simulink model "Quadrotor_simulation"  (R2019a)
settings: Solver=ode4  StartTime=0.0  StopTime=P.tsim  FixedStep=0.01  RelTol=1e-3
InitFcn:
  | Parameters
undefined symbols (not defined in the file or in its folder): Att_Head_PD_ctrl, Att_heading_MST_SMC, Att_heading_SMC, Dist_att, Dist_att2, Dist_pos, E_Kalman_Filter, GPS, IMU, LPF, LPF_F, P, Position_MST_SMC, Position_PD_Ctrl, Position_SMC, Quad_states_plot, Quadrotor_draw, Trajectory
settings Model: Creator=Hp_lap  LastModifiedBy=User
settings SolverCC: AlgebraicLoopSolver=LineSearch
settings DataIOCC: SaveFormat=Array  SaveState=on  DSMLogging=off  ReturnWorkspaceOutputs=off  LoggingToFile=on

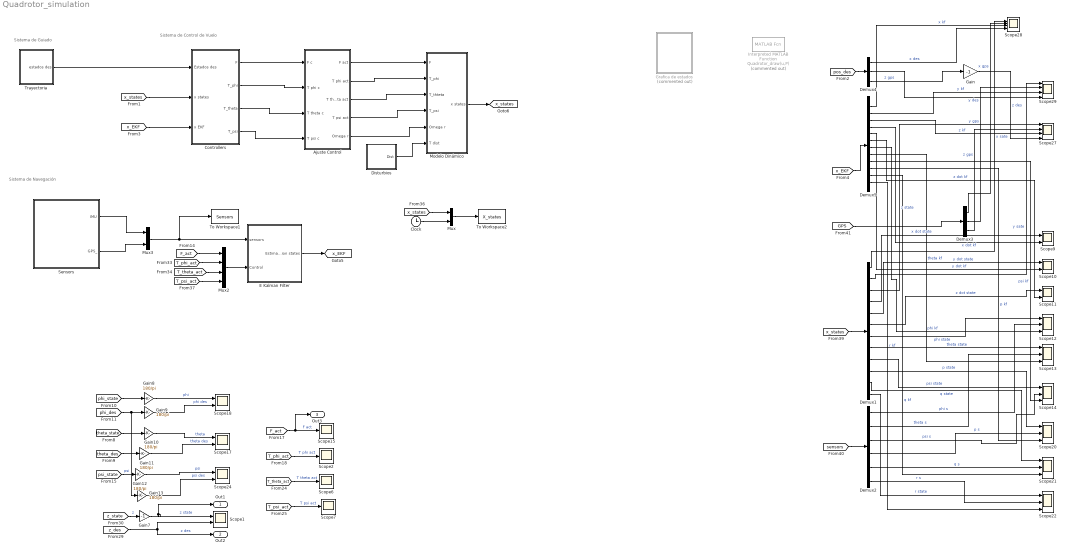
== system Quadrotor_simulation ==
  note: Sistema de Navegación
  note: Sistema de Control de Vuelo
  note: Sistema de Guiado
  Ajuste Control : Subsystem
  Clock : Clock
  Controllers : Subsystem
  Demux1 : Demux  Outputs=12
  Demux2 : Demux  Outputs=6
  Demux3 : Demux  Outputs=3
  Demux4 : Demux  Outputs=3
  Demux5 : Demux  Outputs=12
  Disturbios : Subsystem
  E Kalman Filter : Subsystem
  Gain : Gain  Gain=-1
  Gain{8..13} (6 alike) : Gain  Gain=180/pi
  Gain7 : Gain  Gain=-1
  Grafica de estados : Subsystem  Commented=on
  Interpreted MATLAB Function : MATLABFcn  Commented=on  MATLABFcn=Quadrotor_draw(u,P)  OutputDimensions=0  SampleTime=0.1
  Modelo Dinámico : Subsystem
  Mux : Mux  Inputs=2
  Mux2 : Mux
  Mux3 : Mux  Inputs=2
  Scope{1,9..11,17..18,24} (7 alike) : Scope  NumInputPorts=2
  Scope{12..14,20..22} (6 alike) : Scope  NumInputPorts=3
  Scope{2,6..7,15} (4 alike) : Scope
  Scope27 : Scope  NumInputPorts=4
  Scope28 : Scope  NumInputPorts=4
  Scope29 : Scope  NumInputPorts=4
  Sensors : Subsystem
  To Workspace1 : ToWorkspace  VariableName=Sensors  SampleTime=0.01
  To Workspace2 : ToWorkspace  VariableName=X_states  SampleTime=0.01
  Trayectoria : Subsystem
  Out1 : Outport
  Out2 : Outport  Port=2
  Out3 : Outport  Port=3
  tag scope: x_EKF=global, x_states=global
  wires:
  Mux/1 -> To Workspace2/1
  Clock/1 -> Mux/2
  Disturbios/1(Dist) -> Modelo Dinámico/6(T dist)
  [x_states] -> Mux/1
  Demux5/1 -> Scope28/3  "x kf"
  Demux5/2 -> Scope29/3  "y kf"
  Demux5/3 -> Scope27/3  "z kf"
  Demux5/4 -> Scope9/2  "x dot kf"
  Demux5/5 -> Scope10/2  "y dot kf"
  Demux5/6 -> Scope11/2  "z dot kf"
  Demux5/10 -> Scope20/3  "p kf"
  Demux5/11 -> Scope21/3  "q kf"
  Demux5/12 -> Scope22/3  "r kf"
  [GPS] -> Demux3/1
  Demux1/3 -> Scope27/1  "z state"
  Demux1/1 -> Scope28/1  "x sate"
  Demux3/1 -> Scope28/2  "x gps"
  Demux1/2 -> Scope29/1  "y sate"
  Demux3/2 -> Scope29/2  "y gps"
  Demux3/3 -> Scope27/2  "z gps"
  [x_states] -> Demux1/1
  [sensors] -> Demux2/1
  Demux1/4 -> Scope9/1  "x dot state"
  Demux1/5 -> Scope10/1  "y dot state"
  Demux1/6 -> Scope11/1  "z dot state"
  Demux1/7 -> Scope12/1  "phi state"
  Demux5/7 -> Scope12/3  "phi kf"
  Demux2/1 -> Scope12/2  "phi s"
  Demux1/8 -> Scope13/1  "theta state"
  Demux2/2 -> Scope13/2  "theta s"
  Demux1/9 -> Scope14/1  "psi state"
  Demux2/3 -> Scope14/2  "psi s"
  Demux5/8 -> Scope13/3  "theta kf"
  Demux5/9 -> Scope14/3  "psi kf"
  Demux1/10 -> Scope20/1  "p state"
  Demux2/4 -> Scope20/2  "p s"
  Demux1/11 -> Scope21/1  "q state"
  Demux2/5 -> Scope21/2  "q s"
  Demux1/12 -> Scope22/1  "r state"
  Demux2/6 -> Scope22/2  "r s"
  Modelo Dinámico/1(x states) -> [x_states]
  [pos_des] -> Demux4/1
  Demux4/3 -> Gain/1  "z gps"
  Gain/1 -> Scope27/4  "z des"
  Demux4/2 -> Scope29/4  "y des"
  Demux4/1 -> Scope28/4  "x des"
  Ajuste Control/5(Omega r) -> Modelo Dinámico/5(Omega r)
  [x_states] -> Controllers/2(" x states")
  [x_EKF] -> Controllers/3(x EKF)
  Gain12/1 -> Scope24/1  "psi"
  [psi_state] -> Gain12/1  "psi"
  [theta_des] -> Gain11/1
  Gain9/1 -> Scope18/2  "phi des"
  [phi_des] -> Gain13/1, Gain9/1
  [theta_state] -> Gain10/1
  Gain11/1 -> Scope17/2  "theta des"
  Gain13/1 -> Scope24/2  "psi des"
  Gain8/1 -> Scope18/1  "phi"
  Gain10/1 -> Scope17/1  "theta"
  [phi_state] -> Gain8/1
  [z_des] -> Scope1/2, Out2/1  "z des"
  Gain7/1 -> Scope1/1, Out1/1  "z state"
  [z_state] -> Gain7/1  "z"
  Controllers/1(F) -> Ajuste Control/1(F c)
  Controllers/2(T_phi) -> Ajuste Control/2(T phi c)
  Controllers/3(T_theta) -> Ajuste Control/3(T theta c)
  Controllers/4(T_psi) -> Ajuste Control/4(T psi c)
  [F_act] -> Out3/1, Scope15/1  "F act"
  [T_phi_act] -> Scope2/1  "T phi act"
  [T_theta_act] -> Scope6/1  "T theta act"
  [T_psi_act] -> Scope7/1  "T psi act"
  Ajuste Control/1(F act) -> Modelo Dinámico/1(F)
  Ajuste Control/2(T phi act) -> Modelo Dinámico/2(T_phi)
  Ajuste Control/3(T theta act) -> Modelo Dinámico/3(T_thteta)
  Ajuste Control/4(T psi act) -> Modelo Dinámico/4(T_psi)
  [T_phi_act] -> Mux2/2
  [F_act] -> Mux2/1
  Sensors/2(GPS_) -> Mux3/2
  Sensors/1(IMU) -> Mux3/1
  [T_psi_act] -> Mux2/4
  E Kalman Filter/1(Estimation states) -> [x_EKF]
  [T_theta_act] -> Mux2/3
  Mux2/1 -> E Kalman Filter/2(Control)
  Mux3/1 -> To Workspace1/1, E Kalman Filter/1(sensors)
  [x_EKF] -> Demux5/1
  Trayectoria/1("\testados des") -> Controllers/1(Estados des)

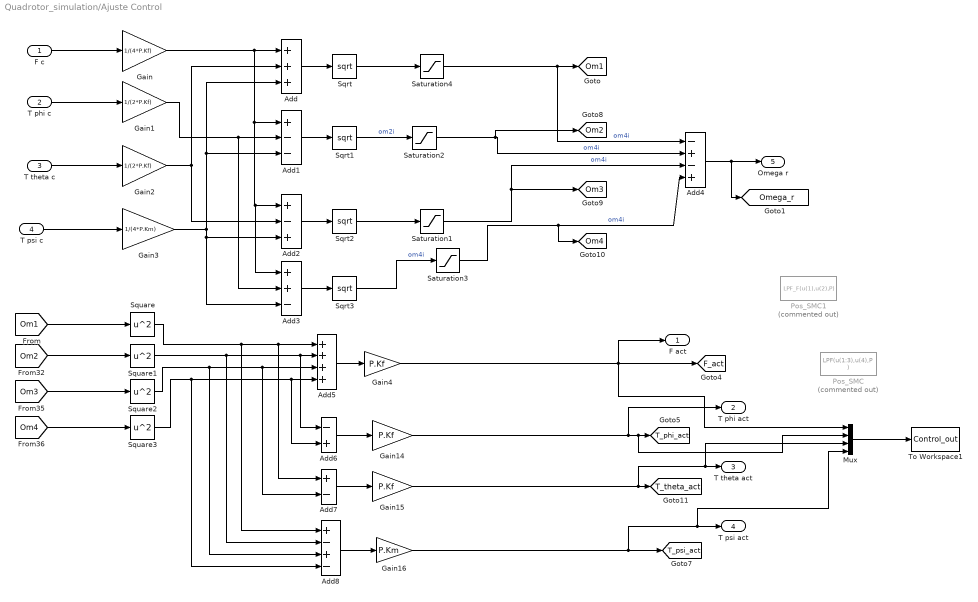
== system Quadrotor_simulation/Ajuste Control ==
  F c : Inport
  T phi c : Inport  Port=2
  T theta c : Inport  Port=3
  T psi c : Inport  Port=4
  Add : Sum  Inputs=+++
  Add1 : Sum  Inputs=+--
  Add2 : Sum  Inputs=+-+
  Add3 : Sum  Inputs=++-
  Add4 : Sum  Inputs=-+-+
  Add5 : Sum  Inputs=++++
  Add6 : Sum  Inputs=-+
  Add7 : Sum  Inputs=+-
  Add8 : Sum  Inputs=+-+-
  Gain : Gain  Gain=1/(4*P.Kf)
  Gain1 : Gain  Gain=1/(2*P.Kf)
  Gain14 : Gain  Gain=P.Kf
  Gain15 : Gain  Gain=P.Kf
  Gain16 : Gain  Gain=P.Km
  Gain2 : Gain  Gain=1/(2*P.Kf)
  Gain3 : Gain  Gain=1/(4*P.Km)
  Gain4 : Gain  Gain=P.Kf
  Mux : Mux
  Pos_SMC : MATLABFcn  Commented=on  MATLABFcn=LPF(u(1:3),u(4),P )  OutputDimensions=3  SampleTime=0.01
  Pos_SMC1 : MATLABFcn  Commented=on  MATLABFcn=LPF_F(u(1),u(2),P)  OutputDimensions=1  SampleTime=0.01
  Saturation{1..4} (4 alike) : Saturate  UpperLimit=435  LowerLimit=0
  Sqrt{,1..3} (4 alike) : Sqrt  OutputSignalType=real  SaturateOnIntegerOverflow=on
  Square{,1..3} (4 alike) : Math  Operator=square  SaturateOnIntegerOverflow=on
  To Workspace1 : ToWorkspace  VariableName=Control_out  SampleTime=0.01
  F act : Outport
  T phi act : Outport  Port=2
  T theta act : Outport  Port=3
  T psi act : Outport  Port=4
  Omega r : Outport  Port=5
  tag scope: F_act=global, Om1=global, Om2=global, Om3=global, Om4=global, Omega_r=global, T_phi_act=global, T_psi_act=global, T_theta_act=global
  wires:
  Add4/1 -> [Omega_r], Omega r/1
  Square2/1 -> Add8/3, Add7/2, Add5/3
  Add8/1 -> Gain16/1
  Gain/1 -> Add/1, Add3/1, Add2/1, Add1/1
  Square/1 -> Add8/1, Add7/1, Add5/1
  Gain1/1 -> Add1/2, Add3/2
  Gain3/1 -> Add3/3, Add2/3, Add1/3, Add/3
  Gain2/1 -> Add2/2, Add/2
  Square1/1 -> Add8/2, Add6/1, Add5/2
  Add/1 -> Sqrt/1
  Add6/1 -> Gain14/1
  Add1/1 -> Sqrt1/1
  Add2/1 -> Sqrt2/1
  [Om1] -> Square/1
  Add5/1 -> Gain4/1
  [Om2] -> Square1/1
  Add3/1 -> Sqrt3/1
  [Om3] -> Square2/1
  Square3/1 -> Add8/4, Add6/2, Add5/4
  Add7/1 -> Gain15/1
  [Om4] -> Square3/1
  Mux/1 -> To Workspace1/1
  Gain16/1 -> Mux/4, T psi act/1, [T_psi_act]
  Gain15/1 -> Mux/3, T theta act/1, [T_theta_act]
  Gain14/1 -> T phi act/1, Mux/2, [T_phi_act]
  Gain4/1 -> F act/1, [F_act], Mux/1
  Sqrt3/1 -> Saturation3/1  "om4i"
  Saturation3/1 -> [Om4], Add4/4  "om4i"
  Sqrt2/1 -> Saturation1/1
  Saturation1/1 -> Add4/3, [Om3]  "om4i"
  Sqrt1/1 -> Saturation2/1  "om2i"
  Saturation2/1 -> [Om2], Add4/2  "om4i"
  Sqrt/1 -> Saturation4/1
  Saturation4/1 -> Add4/1, [Om1]  "om4i"
  F c/1 -> Gain/1
  T phi c/1 -> Gain1/1
  T theta c/1 -> Gain2/1
  T psi c/1 -> Gain3/1

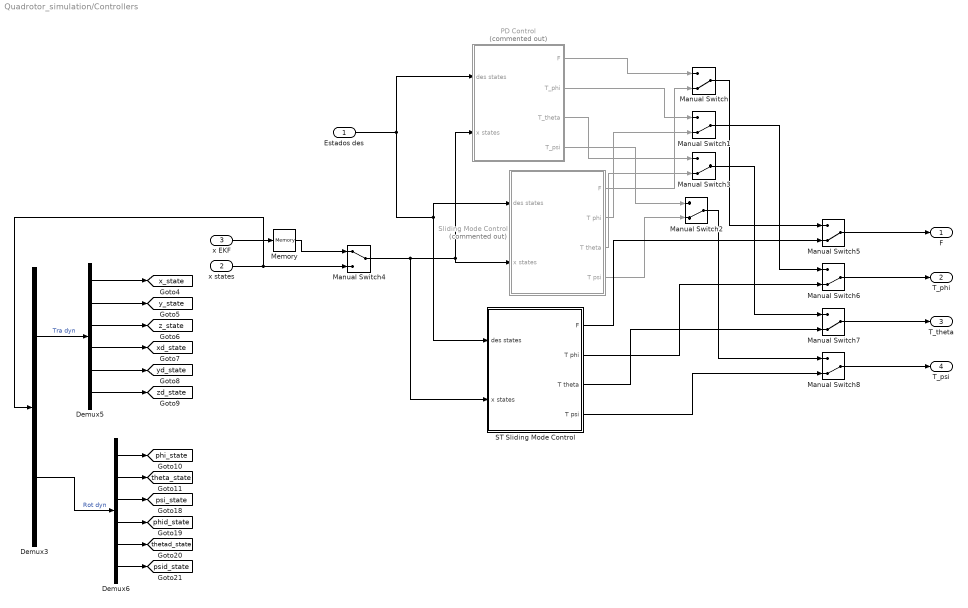
== system Quadrotor_simulation/Controllers ==
  Estados des : Inport
  " x states" : Inport  Port=2
  x EKF : Inport  Port=3
  Demux3 : Demux  Outputs=2
  Demux5 : Demux  Outputs=6
  Demux6 : Demux  Outputs=6
  Manual Switch{,1..3,5..8} (8 alike) : ManualSwitch  CurrentSetting=0
  Manual Switch4 : ManualSwitch
  Memory : Memory  InitialCondition=[P.x0;P.y0;P.z0;P.x0_dot;P.y0_dot;P.z0_dot;P.phi0;P.theta0;P.psi0;P.phi0_dot;P.theta0_dot;P.psi0_dot]  LinearizeMemory=on  LinearizeAsDelay=on
  PD Control : Subsystem  Commented=on
  "ST Sliding Mode Control " : Subsystem
  "Sliding Mode Control " : Subsystem  Commented=on
  F : Outport
  T_phi : Outport  Port=2
  T_theta : Outport  Port=3
  T_psi : Outport  Port=4
  tag scope: phi_state=global, phid_state=global, psi_state=global, psid_state=global, theta_state=global, thetad_state=global, x_state=global, xd_state=global, y_state=global, yd_state=global, z_state=global, zd_state=global
  wires:
  "Sliding Mode Control "/1(F) -> Manual Switch/2
  "Sliding Mode Control "/2(T phi) -> Manual Switch1/2
  "Sliding Mode Control "/3(T theta) -> Manual Switch3/2
  "Sliding Mode Control "/4(T psi) -> Manual Switch2/2
  x EKF/1 -> Memory/1
  Manual Switch4/1 -> "ST Sliding Mode Control "/2(x states), "Sliding Mode Control "/2(x states), PD Control/2(x states)
  Memory/1 -> Manual Switch4/1
  Estados des/1 -> PD Control/1(des states), "ST Sliding Mode Control "/1(des states), "Sliding Mode Control "/1(des states)
  PD Control/1(F) -> Manual Switch/1
  PD Control/2(T_phi) -> Manual Switch1/1
  PD Control/3(T_theta) -> Manual Switch3/1
  PD Control/4(T_psi) -> Manual Switch2/1
  Manual Switch/1 -> Manual Switch5/1
  Manual Switch1/1 -> Manual Switch6/1
  Manual Switch3/1 -> Manual Switch7/1
  Manual Switch2/1 -> Manual Switch8/1
  Demux5/6 -> [zd_state]
  Demux6/6 -> [psid_state]
  Demux6/5 -> [thetad_state]
  Demux6/4 -> [phid_state]
  Demux3/1 -> Demux5/1  "Tra dyn"
  Demux3/2 -> Demux6/1  "Rot dyn"
  Demux6/3 -> [psi_state]
  Demux5/1 -> [x_state]
  Demux5/3 -> [z_state]
  Demux6/2 -> [theta_state]
  Demux5/2 -> [y_state]
  Demux5/5 -> [yd_state]
  Demux5/4 -> [xd_state]
  " x states"/1 -> Demux3/1, Manual Switch4/2
  Demux6/1 -> [phi_state]
  "ST Sliding Mode Control "/1(F) -> Manual Switch5/2
  "ST Sliding Mode Control "/2(T phi) -> Manual Switch6/2
  "ST Sliding Mode Control "/3(T theta) -> Manual Switch7/2
  "ST Sliding Mode Control "/4(T psi) -> Manual Switch8/2
  Manual Switch5/1 -> F/1
  Manual Switch6/1 -> T_phi/1
  Manual Switch7/1 -> T_theta/1
  Manual Switch8/1 -> T_psi/1

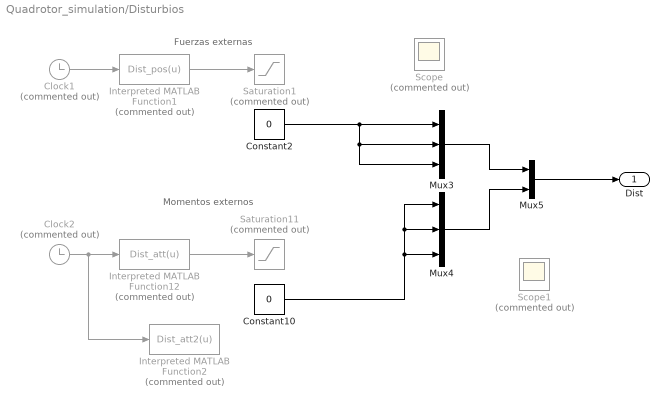
== system Quadrotor_simulation/Disturbios ==
  note: Momentos externos
  note: Fuerzas externas
  Clock1 : Clock  Commented=on
  Clock2 : Clock  Commented=on
  Constant10 : Constant  Value=0
  Constant2 : Constant  Value=0
  Interpreted MATLAB Function1 : MATLABFcn  Commented=on  MATLABFcn=Dist_pos(u)  OutputDimensions=1  SampleTime=0.01
  Interpreted MATLAB Function12 : MATLABFcn  Commented=on  MATLABFcn=Dist_att(u)  OutputDimensions=1  SampleTime=0.01
  Interpreted MATLAB Function2 : MATLABFcn  Commented=on  MATLABFcn=Dist_att2(u)  OutputDimensions=1  SampleTime=0.01
  Mux3 : Mux  Inputs=3
  Mux4 : Mux  Inputs=3
  Mux5 : Mux  Inputs=2
  Saturation1 : Saturate  Commented=on
  Saturation11 : Saturate  Commented=on  UpperLimit=0.25  LowerLimit=-0.25
  Scope : Scope  Commented=on
  Scope1 : Scope  Commented=on
  Dist : Outport
  wires:
  Interpreted MATLAB Function12/1 -> Saturation11/1
  Mux3/1 -> Mux5/1
  Mux4/1 -> Mux5/2
  Mux5/1 -> Dist/1
  Clock2/1 -> Interpreted MATLAB Function2/1, Interpreted MATLAB Function12/1
  Interpreted MATLAB Function1/1 -> Saturation1/1
  Clock1/1 -> Interpreted MATLAB Function1/1
  Constant2/1 -> Mux3/3, Mux3/2, Mux3/1
  Constant10/1 -> Mux4/3, Mux4/2, Mux4/1

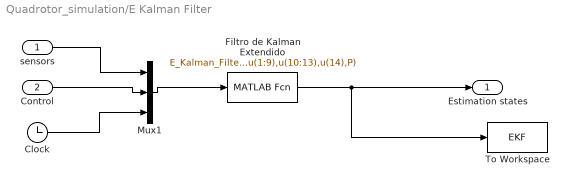
== system Quadrotor_simulation/E Kalman Filter ==
  sensors : Inport
  Control : Inport  Port=2
  Clock : Clock
  Filtro de Kalman Extendido : MATLABFcn  MATLABFcn=E_Kalman_Filter(u(1:9),u(10:13),u(14),P)  OutputDimensions=12  SampleTime=0.01
  Mux1 : Mux  Inputs=3
  To Workspace : ToWorkspace  VariableName=EKF  SampleTime=0.01
  Estimation states : Outport
  wires:
  Mux1/1 -> Filtro de Kalman Extendido/1
  Clock/1 -> Mux1/3
  Control/1 -> Mux1/2
  sensors/1 -> Mux1/1
  Filtro de Kalman Extendido/1 -> To Workspace/1, Estimation states/1

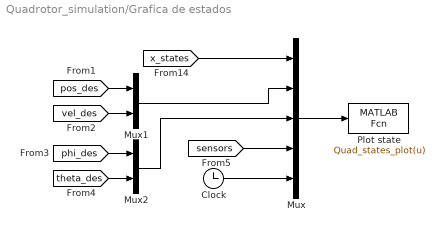
== system Quadrotor_simulation/Grafica de estados ==
  Clock : Clock
  Mux : Mux  Inputs=5
  Mux1 : Mux  Inputs=2
  Mux2 : Mux  Inputs=2
  Plot state : MATLABFcn  MATLABFcn=Quad_states_plot(u)  OutputDimensions=0  SampleTime=0.1
  wires:
  Mux/1 -> Plot state/1
  [x_states] -> Mux/1
  [vel_des] -> Mux1/2
  [pos_des] -> Mux1/1
  Mux1/1 -> Mux/2
  [theta_des] -> Mux2/2
  [phi_des] -> Mux2/1
  Mux2/1 -> Mux/3
  [sensors] -> Mux/4
  Clock/1 -> Mux/5

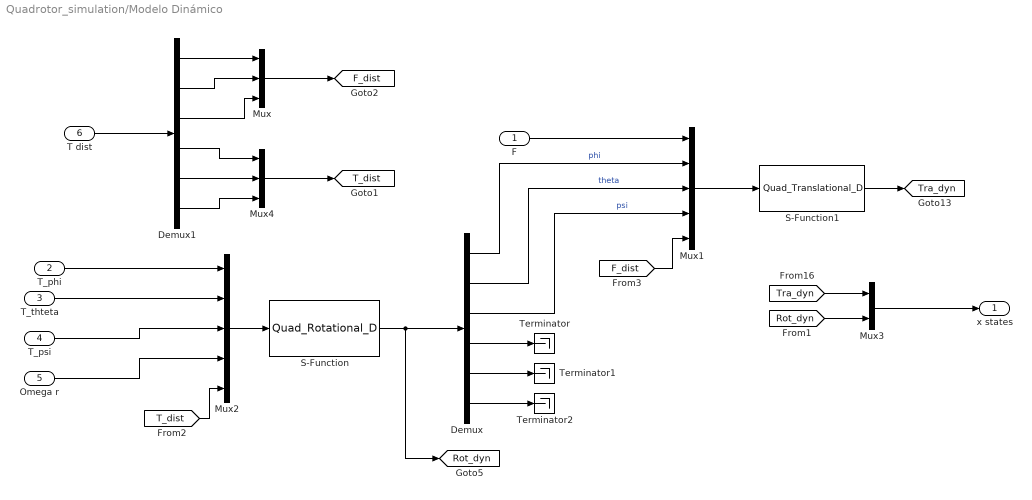
== system Quadrotor_simulation/Modelo Dinámico ==
  F : Inport
  T_phi : Inport  Port=2
  T_thteta : Inport  Port=3
  T_psi : Inport  Port=4
  Omega r : Inport  Port=5
  T dist : Inport  Port=6
  Demux : Demux  Outputs=6
  Demux1 : Demux  Outputs=6
  Mux : Mux  Inputs=3
  Mux1 : Mux  Inputs=5
  Mux2 : Mux  Inputs=5
  Mux3 : Mux  Inputs=2
  Mux4 : Mux  Inputs=3
  S-Function : S-Function  FunctionName=Quad_Rotational_D  Parameters=P  SFunctionDeploymentMode=off  EnableBusSupport=off
  S-Function1 : S-Function  InitFcn=Parameters  FunctionName=Quad_Translational_D  Parameters=P  SFunctionDeploymentMode=off  EnableBusSupport=off
  Terminator : Terminator
  Terminator1 : Terminator
  Terminator2 : Terminator
  x states : Outport
  tag scope: F_dist=global, Rot_dyn=global, T_dist=global, Tra_dyn=global
  wires:
  Mux1/1 -> S-Function1/1
  Mux2/1 -> S-Function/1
  S-Function1/1 -> [Tra_dyn]
  S-Function/1 -> [Rot_dyn], Demux/1
  Demux/2 -> Mux1/3  "theta"
  Demux/1 -> Mux1/2  "phi"
  Demux/3 -> Mux1/4  "psi"
  Demux/6 -> Terminator2/1
  Demux/5 -> Terminator1/1
  Demux/4 -> Terminator/1
  [Tra_dyn] -> Mux3/1
  [Rot_dyn] -> Mux3/2
  T dist/1 -> Demux1/1
  Demux1/1 -> Mux/1
  Demux1/2 -> Mux/2
  Demux1/3 -> Mux/3
  Demux1/4 -> Mux4/1
  Demux1/5 -> Mux4/2
  Demux1/6 -> Mux4/3
  Mux/1 -> [F_dist]
  Mux4/1 -> [T_dist]
  [T_dist] -> Mux2/5
  [F_dist] -> Mux1/5
  F/1 -> Mux1/1
  T_phi/1 -> Mux2/1
  T_thteta/1 -> Mux2/2
  T_psi/1 -> Mux2/3
  Omega r/1 -> Mux2/4
  Mux3/1 -> x states/1

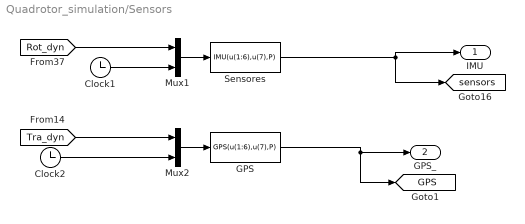
== system Quadrotor_simulation/Sensors ==
  Clock1 : Clock
  Clock2 : Clock
  GPS : MATLABFcn  MATLABFcn=GPS(u(1:6),u(7),P)  OutputDimensions=3  SampleTime=P.Ts_gps
  Mux1 : Mux  Inputs=2
  Mux2 : Mux  Inputs=2
  Sensores : MATLABFcn  MATLABFcn=IMU(u(1:6),u(7),P)  OutputDimensions=6  SampleTime=0.01
  IMU : Outport
  GPS_ : Outport  Port=2
  tag scope: GPS=global, sensors=global
  wires:
  Clock1/1 -> Mux1/2
  Mux1/1 -> Sensores/1
  Mux2/1 -> GPS/1
  Clock2/1 -> Mux2/2
  Sensores/1 -> IMU/1, [sensors]
  GPS/1 -> [GPS], GPS_/1
  [Rot_dyn] -> Mux1/1
  [Tra_dyn] -> Mux2/1

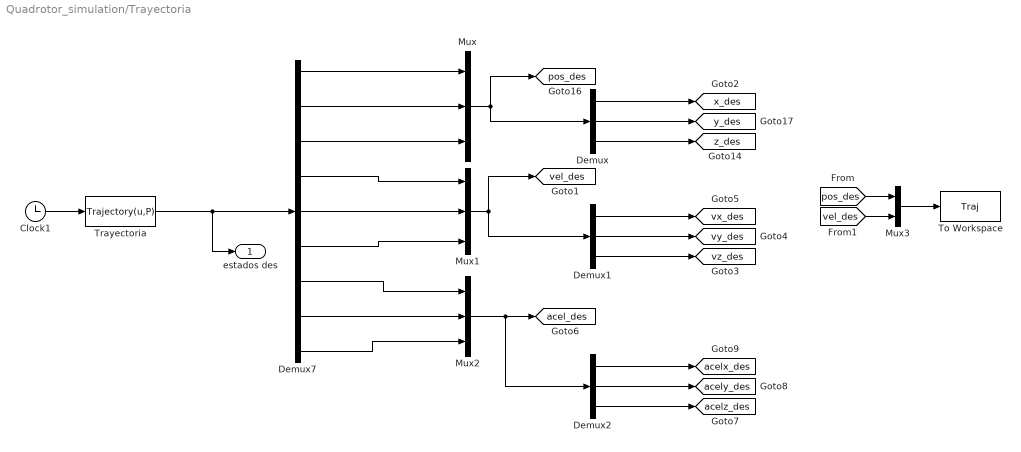
== system Quadrotor_simulation/Trayectoria ==
  Clock1 : Clock
  Demux : Demux  Outputs=3
  Demux1 : Demux  Outputs=3
  Demux2 : Demux  Outputs=3
  Demux7 : Demux  Outputs=9
  Mux : Mux  Inputs=3
  Mux1 : Mux  Inputs=3
  Mux2 : Mux  Inputs=3
  Mux3 : Mux  Inputs=2
  To Workspace : ToWorkspace  VariableName=Traj  SampleTime=0.01
  Trayectoria : MATLABFcn  MATLABFcn=Trajectory(u,P)  OutputDimensions=9  SampleTime=0.01
  "\testados des" : Outport
  tag scope: acel_des=global, acelx_des=global, acely_des=global, acelz_des=global, pos_des=global, vel_des=global, vx_des=global, vy_des=global, vz_des=global, x_des=global, y_des=global, z_des=global
  wires:
  Demux7/6 -> Mux1/3
  Demux7/4 -> Mux1/1
  Clock1/1 -> Trayectoria/1
  Demux7/1 -> Mux/1
  Demux7/5 -> Mux1/2
  Demux7/2 -> Mux/2
  Demux7/3 -> Mux/3
  Demux7/7 -> Mux2/1
  Demux7/8 -> Mux2/2
  Demux7/9 -> Mux2/3
  Mux3/1 -> To Workspace/1
  [pos_des] -> Mux3/1
  [vel_des] -> Mux3/2
  Demux/1 -> [x_des]
  Demux/3 -> [z_des]
  Demux/2 -> [y_des]
  Mux/1 -> Demux/1, [pos_des]
  Mux1/1 -> Demux1/1, [vel_des]
  Demux1/3 -> [vz_des]
  Demux1/2 -> [vy_des]
  Demux1/1 -> [vx_des]
  Demux2/1 -> [acelx_des]
  Mux2/1 -> Demux2/1, [acel_des]
  Demux2/2 -> [acely_des]
  Demux2/3 -> [acelz_des]
  Trayectoria/1 -> "\testados des"/1, Demux7/1

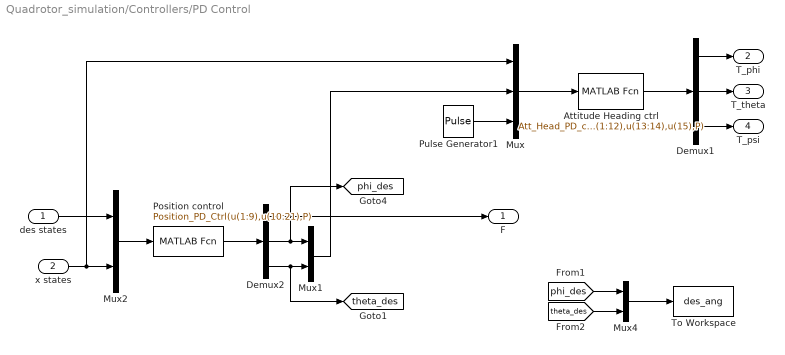
== system Quadrotor_simulation/Controllers/PD Control ==
  des states : Inport
  x states : Inport  Port=2
  Attitude Heading ctrl : MATLABFcn  MATLABFcn=Att_Head_PD_ctrl(u(1:12),u(13:14),u(15),P)  OutputDimensions=3  SampleTime=0.01
  Demux1 : Demux  Outputs=3
  Demux2 : Demux  Outputs=3
  Mux : Mux  Inputs=3
  Mux1 : Mux  Inputs=2
  Mux2 : Mux  Inputs=2
  Mux4 : Mux  Inputs=2
  Position control : MATLABFcn  MATLABFcn=Position_PD_Ctrl(u(1:9),u(10:21),P)  OutputDimensions=3  SampleTime=0.01
  Pulse Generator1 : DiscretePulseGenerator  PulseType=Time based  Amplitude=5*(pi/180)  PulseWidth=50
  To Workspace : ToWorkspace  VariableName=des_ang  SampleTime=0.01
  F : Outport
  T_phi : Outport  Port=2
  T_theta : Outport  Port=3
  T_psi : Outport  Port=4
  tag scope: phi_des=global, theta_des=global
  wires:
  Demux1/1 -> T_phi/1
  Demux1/2 -> T_theta/1
  Demux1/3 -> T_psi/1
  Attitude Heading ctrl/1 -> Demux1/1
  Mux/1 -> Attitude Heading ctrl/1
  Mux2/1 -> Position control/1
  des states/1 -> Mux2/1
  x states/1 -> Mux/1, Mux2/2
  Mux1/1 -> Mux/2
  Demux2/3 -> [theta_des], Mux1/2
  Demux2/1 -> F/1
  Position control/1 -> Demux2/1
  Mux4/1 -> To Workspace/1
  [theta_des] -> Mux4/2
  [phi_des] -> Mux4/1
  Demux2/2 -> [phi_des], Mux1/1
  Pulse Generator1/1 -> Mux/3

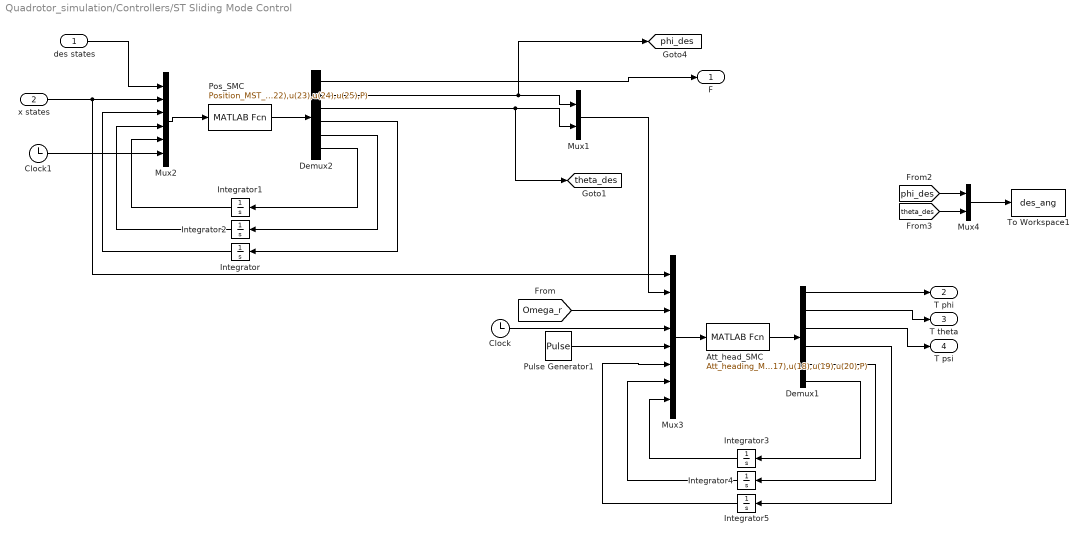
== system Quadrotor_simulation/Controllers/ST Sliding Mode Control  ==
  des states : Inport
  x states : Inport  Port=2
  Att_head_SMC : MATLABFcn  MATLABFcn=Att_heading_MST_SMC(u(1:12),u(13:14),u(15),u(16),u(17),u(18),u(19),u(20),P)  OutputDimensions=6  SampleTime=0.01
  Clock : Clock
  Clock1 : Clock
  Demux1 : Demux  Outputs=6
  Demux2 : Demux  Outputs=6
  Integrator{,1..5} (6 alike) : Integrator
  Mux1 : Mux  Inputs=2
  Mux2 : Mux  Inputs=6
  Mux3 : Mux  Inputs=8
  Mux4 : Mux  Inputs=2
  Pos_SMC : MATLABFcn  MATLABFcn=Position_MST_SMC(u(1:9),u(10:21),u(22),u(23),u(24),u(25),P)  OutputDimensions=6  SampleTime=0.01
  Pulse Generator1 : DiscretePulseGenerator  PulseType=Time based  Amplitude=5*(pi/180)  PulseWidth=50
  To Workspace1 : ToWorkspace  VariableName=des_ang  SampleTime=0.01
  F : Outport
  T phi : Outport  Port=2
  T theta : Outport  Port=3
  T psi : Outport  Port=4
  tag scope: phi_des=global, theta_des=global
  wires:
  Pos_SMC/1 -> Demux2/1
  Mux3/1 -> Att_head_SMC/1
  Att_head_SMC/1 -> Demux1/1
  Demux1/1 -> T phi/1
  Demux1/2 -> T theta/1
  Demux1/3 -> T psi/1
  des states/1 -> Mux2/1
  x states/1 -> Mux3/1, Mux2/2
  Mux2/1 -> Pos_SMC/1
  Demux2/1 -> F/1
  Demux2/2 -> [phi_des], Mux1/1
  Mux1/1 -> Mux3/2
  [Omega_r] -> Mux3/3
  Clock/1 -> Mux3/4
  Pulse Generator1/1 -> Mux3/5
  Demux2/3 -> [theta_des], Mux1/2
  Demux2/4 -> Integrator/1
  Demux2/6 -> Integrator1/1
  Demux2/5 -> Integrator2/1
  Demux1/4 -> Integrator5/1
  Demux1/5 -> Integrator4/1
  Demux1/6 -> Integrator3/1
  Mux4/1 -> To Workspace1/1
  [theta_des] -> Mux4/2
  [phi_des] -> Mux4/1
  Integrator/1 -> Mux2/3
  Integrator2/1 -> Mux2/4
  Integrator1/1 -> Mux2/5
  Integrator5/1 -> Mux3/6
  Integrator4/1 -> Mux3/7
  Integrator3/1 -> Mux3/8
  Clock1/1 -> Mux2/6

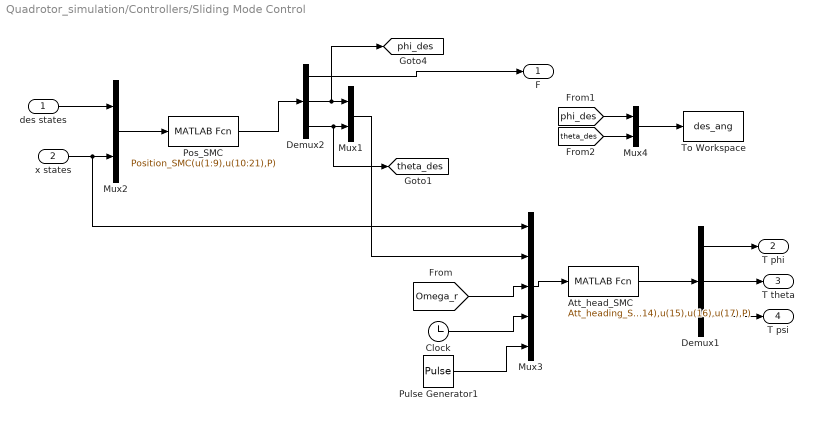
== system Quadrotor_simulation/Controllers/Sliding Mode Control  ==
  des states : Inport
  x states : Inport  Port=2
  Att_head_SMC : MATLABFcn  MATLABFcn=Att_heading_SMC(u(1:12),u(13:14),u(15),u(16),u(17),P)  OutputDimensions=3  SampleTime=0.01
  Clock : Clock
  Demux1 : Demux  Outputs=3
  Demux2 : Demux  Outputs=3
  Mux1 : Mux  Inputs=2
  Mux2 : Mux  Inputs=2
  Mux3 : Mux  Inputs=5
  Mux4 : Mux  Inputs=2
  Pos_SMC : MATLABFcn  MATLABFcn=Position_SMC(u(1:9),u(10:21),P)  OutputDimensions=3  SampleTime=0.01
  Pulse Generator1 : DiscretePulseGenerator  PulseType=Time based  Amplitude=5*(pi/180)  PulseWidth=50
  To Workspace : ToWorkspace  VariableName=des_ang  SampleTime=0.01
  F : Outport
  T phi : Outport  Port=2
  T theta : Outport  Port=3
  T psi : Outport  Port=4
  tag scope: phi_des=global, theta_des=global
  wires:
  Pos_SMC/1 -> Demux2/1
  Mux3/1 -> Att_head_SMC/1
  Att_head_SMC/1 -> Demux1/1
  Demux1/1 -> T phi/1
  Demux1/2 -> T theta/1
  Demux1/3 -> T psi/1
  des states/1 -> Mux2/1
  x states/1 -> Mux3/1, Mux2/2
  Mux2/1 -> Pos_SMC/1
  Demux2/1 -> F/1
  Demux2/2 -> [phi_des], Mux1/1
  Mux1/1 -> Mux3/2
  Demux2/3 -> [theta_des], Mux1/2
  [Omega_r] -> Mux3/3
  Clock/1 -> Mux3/4
  [phi_des] -> Mux4/1
  [theta_des] -> Mux4/2
  Mux4/1 -> To Workspace/1
  Pulse Generator1/1 -> Mux3/5
